simulink model "NR_PDSCH_LinkLevel_Sim"  (R2026a)
settings: Solver=FixedStepDiscrete  StopTime=59  FixedStep=1
InitFcn:
  | addpath(genpath(pwd));
  | if exist('set_sim_profile.m','file'); set_sim_profile('massive'); end
  | cfg = config();
  | assert(cfg.nTx==64 && cfg.nRx==8 && cfg.nLayers==4, ...
  |     'This 64x8 bench needs the massive profile: run set_sim_profile(''massive'')');
  | rng(cfg.randomSeed);
  | run_verification_gates(cfg);   % gates before results
StopFcn:
  | ber = sum(log_bitErrors)/sum(log_nBits);
  | bler = mean(log_blockError);
  | fprintf('\n=== Simulink run aggregate (one SNR point) ===\n');
  | fprintf('BER  = %.5g\nBLER = %.4g\nEVM  = %.4g %%\nNMSE = %.5g\nCapacity = %.4g bit/s/Hz\n', ...
  |     ber, bler, 100*mean(log_evm), mean(log_nmse), mean(log_capacity));
undefined symbols (not defined in the file or in its folder): DiscIntNeverNeededParam
Description:
  | PDSCH-oriented 64x8 Massive MIMO-OFDM link-level test bench, four spatial
  | layers with wideband SVD eigen-beamforming, 144 active subcarriers, 14 OFDM
  | symbols per frame, flat Rayleigh channel. One Monte Carlo frame per step;
  | sixty steps reproduce one SNR point of the massive grid. Every block calls
  | the verified MATLAB chain through thin sl_*.m wrappers; the InitFcn selects
  | the massive profile and runs the verification gates before the first step.
  | Signal dimensions are fixed inside the blocks; rebuilding with
  | build_nr_pdsch_simulink regenerates them from config.m.
settings Model: Creator=mokle  LastModifiedBy=mokle

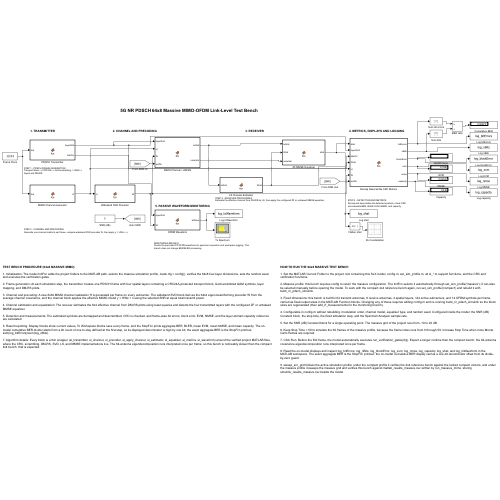
[thumbnail: Simulink's stored preview of the top-level diagram]
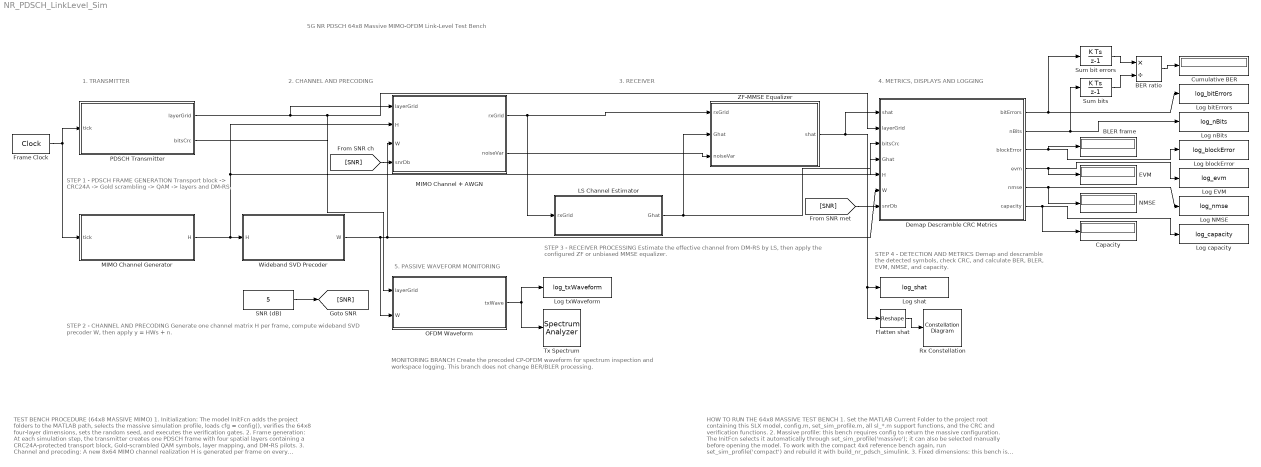
== system NR_PDSCH_LinkLevel_Sim ==
  note: 5G NR PDSCH 64x8 Massive MIMO-OFDM Link-Level Test Bench
  note: 1. TRANSMITTER
  note: 2. CHANNEL AND PRECODING
  note: 3. RECEIVER
  note: 4. METRICS, DISPLAYS AND LOGGING
  note: 5. PASSIVE WAVEFORM MONITORING
  note: STEP 1 - PDSCH FRAME GENERATION
      | Transport block -> CRC24A -> Gold scrambling -> QAM -> layers and DM-RS.
  note: STEP 2 - CHANNEL AND PRECODING
      | Generate one channel matrix H per frame, compute wideband SVD precoder W, then apply y = HWs + n.
  note: STEP 3 - RECEIVER PROCESSING
      | Estimate the effective channel from DM-RS by LS, then apply the configured ZF or unbiased MMSE equalizer.
  note: STEP 4 - DETECTION AND METRICS
      | Demap and descramble the detected symbols, check CRC, and calculate BER, BLER, EVM, NMSE, and capacity.
  note: MONITORING BRANCH
      | Create the precoded CP-OFDM waveform for spectrum inspection and workspace logging. This branch does not change BER/BLER processing.
  note: TEST BENCH PROCEDURE (64x8 MASSIVE MIMO)
      |
      | 1. Initialization: The model InitFcn adds the project folders to the MATLAB path, selects the massive simulation profile, loads cfg = config(), verifies the 64x8 four-layer dimensions, sets the random seed, and executes the verification gates.
      |
      | 2. Frame generation: At each simulation step, the transmitter creates one PDSCH frame with four spatial layers containing a CRC24A-protected transport block, Gold-scrambled QAM symbols, layer mapping, and DM-RS pilots.
      |
      | 3. Channel and precoding: A new 8x64 MIMO channel realization H is generated per frame on every subcarrier. The wideband SVD block derives the 64x4 eigen-beamforming precoder W from the average channel covariance, and the channel block applies the effective MIMO model y = HWs + n using the selected SNR at equal total transmit power.
      |
      | 4. Channel estimation and equalization: The receiver estimates the 8x4 effective channel from DM-RS pilots using least squares and detects the four transmitted layers with the configured ZF or unbiased MMSE equalizer.
      |
      | 5. Detection and measurements: The estimated symbols are demapped and descrambled, CRC is checked, and frame-wise bit errors, block error, EVM, NMSE, and the layer-domain capacity reference are calculated.
      |
      | 6. Result reporting: Display blocks show current values, To Workspace blocks save every frame, and the StopFcn prints aggregate BER, BLER, mean EVM, mean NMSE, and mean capacity. The on-model cumulative BER divider starts from a bit count of one to stay defined at the first step, so its displayed denominator is high by one bit; the exact aggregate BER is the StopFcn printout, sum(log_bitErrors)/sum(log_nBits).
      |
      | 7. Algorithm details: Every block is a thin wrapper (sl_transmitter, sl_channel, sl_precoder, sl_apply_channel, sl_estimator, sl_equalizer, sl_metrics, sl_waveform) around the verified project MATLAB files, where the CRC, scrambling, DM-RS, SVD, LS, and MMSE implementations live. The 64-antenna eigendecomposition runs interpreted once per frame, so this bench is noticeably slower than the compact 4x4 bench; that is expected.
  note: HOW TO RUN THE 64x8 MASSIVE TEST BENCH
      |
      | 1. Set the MATLAB Current Folder to the project root containing this SLX model, config.m, set_sim_profile.m, all sl_*.m support functions, and the CRC and verification functions.
      |
      | 2. Massive profile: this bench requires config to return the massive configuration. The InitFcn selects it automatically through set_sim_profile('massive'); it can also be selected manually before opening the model. To work with the compact 4x4 reference bench again, run set_sim_profile('compact') and rebuild it with build_nr_pdsch_simulink.
      |
      | 3. Fixed dimensions: this bench is built for 64 transmit antennas, 8 receive antennas, 4 spatial layers, 144 active subcarriers, and 14 OFDM symbols per frame, carried as fixed output sizes in the MATLAB Function blocks. Changing any of these requires editing config.m and re-running build_nr_pdsch_simulink so the block sizes are regenerated (then add_rf_measurements for the monitoring branch).
      |
      | 4. Configurable in config.m without rebuilding: modulation order, channel model, equalizer type, and random seed. Configured inside the model: the SNR (dB) Constant block, the stop time, the fixed simulation step, and the Spectrum Analyzer sample rate.
      |
      | 5. Set the SNR (dB) Constant block for a single operating point. The massive grid of the project runs from -10 to 20 dB.
      |
      | 6. Keep Stop Time = 59 to simulate the 60 frames of the massive profile, because the frame index runs from 0 through 59. Increase Stop Time when more Monte Carlo frames are required.
      |
      | 7. Click Run. Before the first frame, the model automatically executes run_verification_gates(cfg). Expect a longer runtime than the compact bench: the 64-antenna covariance eigendecomposition runs interpreted once per frame.
      |
      | 8. Read the on-model displays and inspect log_bitErrors, log_nBits, log_blockError, log_evm, log_nmse, log_capacity, log_shat, and log_txWaveform in the MATLAB workspace. The exact aggregate BER is the StopFcn printout; the on-model cumulative BER display carries a one-bit denominator offset from its divide-by-zero guard.
      |
      | 9. sweep_snr_grid follows the active simulation profile: under the compact profile it verifies the 4x4 reference bench against the locked compact vectors, and under the massive profile it sweeps the massive grid and verifies this bench against matlab_results_massive.csv written by run_massive_mimo, storing simulink_results_massive.csv beside the model.
  BER ratio : Product  Inputs=*/
  BLER frame : Display
  Capacity : Display
  Cumulative BER : Display
  Demap Descramble CRC Metrics : MATLAB Function  TreatAsAtomicUnit=on
  EVM : Display
  Flatten shat : Reshape
  Frame Clock : DigitalClock
  LS Channel Estimator : MATLAB Function  TreatAsAtomicUnit=on
  Log EVM : ToWorkspace  VariableName=log_evm  SampleTime=-1
  Log NMSE : ToWorkspace  VariableName=log_nmse  SampleTime=-1
  Log bitErrors : ToWorkspace  VariableName=log_bitErrors  SampleTime=-1
  Log blockError : ToWorkspace  VariableName=log_blockError  SampleTime=-1
  Log capacity : ToWorkspace  VariableName=log_capacity  SampleTime=-1
  Log nBits : ToWorkspace  VariableName=log_nBits  SampleTime=-1
  Log shat : ToWorkspace  VariableName=log_shat  SampleTime=-1
  Log txWaveform : ToWorkspace  VariableName=log_txWaveform  SampleTime=-1
  MIMO Channel + AWGN : MATLAB Function  TreatAsAtomicUnit=on
  MIMO Channel Generator : MATLAB Function  TreatAsAtomicUnit=on
  NMSE : Display
  OFDM Waveform : MATLAB Function  TreatAsAtomicUnit=on
  PDSCH Transmitter : MATLAB Function  TreatAsAtomicUnit=on
  Rx Constellation : ConstellationDiagram  WindowPosition=[3047.000000,241.000000,600.000000,671.000000,]  ScopeFrameLocation=window  ReferenceConstellation=[-0.948683-0.948683i -0.948683-0.316228i -0.948683+0.316228i -0.948683+0.948683i -0.316228-0.948683i -0.316228-0.316228i -0.316228+0.316228i -0.316228+0.948683i 0.316228-0.948683i 0.316228-0.316228i 0.316228+0.316228i 0.316228+0.948683i 0.948683-0.948683i 0.948683-0.316228i 0.948683+0.316228i 0.948683+0.948683i]
  SNR (dB) : Constant  Value=5  SampleTime=1
  Sum bit errors : DiscreteIntegrator  ICPrevOutput=DiscIntNeverNeededParam  ICPrevScaledInput=DiscIntNeverNeededParam
  Sum bits : DiscreteIntegrator  InitialCondition=1  ICPrevOutput=DiscIntNeverNeededParam  ICPrevScaledInput=DiscIntNeverNeededParam
  Tx Spectrum : SpectrumAnalyzer  WindowPosition=[2247.000000,243.000000,800.000000,668.000000,]  ScopeFrameLocation=window  SampleRateSource=Property  SampleRate=7680000  WindowInvariantSamplesPerUpdate=on  YLimits=[-50.9635 -3.836]
  Wideband SVD Precoder : MATLAB Function  TreatAsAtomicUnit=on
  ZF-MMSE Equalizer : MATLAB Function  TreatAsAtomicUnit=on
  wires:
  Frame Clock/1 -> PDSCH Transmitter/1(tick), MIMO Channel Generator/1(tick)
  SNR (dB)/1 -> [SNR]
  PDSCH Transmitter/1(layerGrid) -> Demap Descramble CRC Metrics/2(layerGrid), OFDM Waveform/1(layerGrid), MIMO Channel + AWGN/1(layerGrid)
  MIMO Channel Generator/1(H) -> MIMO Channel + AWGN/2(H), Demap Descramble CRC Metrics/5(H), Wideband SVD Precoder/1(H)
  Wideband SVD Precoder/1(W) -> MIMO Channel + AWGN/3(W), Demap Descramble CRC Metrics/6(W), OFDM Waveform/2(W)
  [SNR] -> MIMO Channel + AWGN/4(snrDb)
  MIMO Channel + AWGN/1(rxGrid) -> LS Channel Estimator/1(rxGrid), ZF-MMSE Equalizer/1(rxGrid)
  LS Channel Estimator/1(Ghat) -> ZF-MMSE Equalizer/2(Ghat), Demap Descramble CRC Metrics/4(Ghat)
  MIMO Channel + AWGN/2(noiseVar) -> ZF-MMSE Equalizer/3(noiseVar)
  ZF-MMSE Equalizer/1(shat) -> Log shat/1, Flatten shat/1, Demap Descramble CRC Metrics/1(shat)
  PDSCH Transmitter/2(bitsCrc) -> Demap Descramble CRC Metrics/3(bitsCrc)
  [SNR] -> Demap Descramble CRC Metrics/7(snrDb)
  Demap Descramble CRC Metrics/1(bitErrors) -> Sum bit errors/1, Log bitErrors/1
  Demap Descramble CRC Metrics/2(nBits) -> Sum bits/1, Log nBits/1
  Sum bit errors/1 -> BER ratio/1
  Sum bits/1 -> BER ratio/2
  BER ratio/1 -> Cumulative BER/1
  Demap Descramble CRC Metrics/3(blockError) -> BLER frame/1, Log blockError/1
  Demap Descramble CRC Metrics/4(evm) -> EVM/1, Log EVM/1
  Demap Descramble CRC Metrics/5(nmse) -> NMSE/1, Log NMSE/1
  Demap Descramble CRC Metrics/6(capacity) -> Capacity/1, Log capacity/1
  OFDM Waveform/1(txWave) -> Log txWaveform/1, Tx Spectrum/1
  Flatten shat/1 -> Rx Constellation/1

== matlab function NR_PDSCH_LinkLevel_Sim/MIMO Channel Generator ==
  data: tick input; H output
function H = fcn(tick) %#ok<INUSD>
% generate_channel: one realization per frame (AWGN/Rayleigh/Rician/TDL)
coder.extrinsic('sl_channel');
H = complex(zeros(144,8,64));
H = sl_channel(tick);

== matlab function NR_PDSCH_LinkLevel_Sim/PDSCH Transmitter ==
  data: tick input; layerGrid output; bitsCrc output
function [layerGrid, bitsCrc] = fcn(tick) %#ok<INUSD>
% build_frame: TB -> CRC24A -> Gold scrambling -> QAM -> layers + DM-RS
coder.extrinsic('sl_transmitter');
layerGrid = complex(zeros(14,144,4));
bitsCrc = zeros(27648,1);
[layerGrid, bitsCrc] = sl_transmitter(tick);

== matlab function NR_PDSCH_LinkLevel_Sim/Wideband SVD Precoder ==
  data: H input; W output
function W = fcn(H)
% compute_precoder: wideband eigenbeamforming, eq. (31)
coder.extrinsic('sl_precoder');
W = complex(zeros(64,4));
W = sl_precoder(H);

== matlab function NR_PDSCH_LinkLevel_Sim/MIMO Channel + AWGN ==
  data: layerGrid input; rxGrid output; H input; W input; snrDb input; noiseVar output
function [rxGrid, noiseVar] = fcn(layerGrid, H, W, snrDb)
% apply_mimo_channel: y = HWs + n, eq. (34), total-transmit-SNR noise
coder.extrinsic('sl_apply_channel');
rxGrid = complex(zeros(14,144,8));
noiseVar = 0;
[rxGrid, noiseVar] = sl_apply_channel(layerGrid, H, W, snrDb);

== matlab function NR_PDSCH_LinkLevel_Sim/LS Channel Estimator ==
  data: rxGrid input; Ghat output
function Ghat = fcn(rxGrid)
% estimate_effective_channel_ls: LS on DM-RS, eq. (65)
coder.extrinsic('sl_estimator');
Ghat = complex(zeros(144,8,4));
Ghat = sl_estimator(rxGrid);

== matlab function NR_PDSCH_LinkLevel_Sim/ZF-MMSE Equalizer ==
  data: rxGrid input; shat output; Ghat input; noiseVar input
function shat = fcn(rxGrid, Ghat, noiseVar)
% equalize_mimo: ZF eq. (38) or unbiased MMSE eq. (39), per config.m
coder.extrinsic('sl_equalizer');
shat = complex(zeros(1728,4));
shat = sl_equalizer(rxGrid, Ghat, noiseVar);

== matlab function NR_PDSCH_LinkLevel_Sim/Demap Descramble CRC Metrics ==
  data: shat input; bitErrors output; layerGrid input; bitsCrc input; Ghat input; H input; W input; snrDb input; nBits output; blockError output; evm output; nmse output; capacity output
function [bitErrors, nBits, blockError, evm, nmse, capacity] = fcn(shat, layerGrid, bitsCrc, Ghat, H, W, snrDb)
% compute_frame_metrics: BER (41), BLER (42), EVM (43), NMSE (78), C (110)
coder.extrinsic('sl_metrics');
bitErrors = 0; nBits = 0; blockError = 0; evm = 0; nmse = 0; capacity = 0;
[bitErrors, nBits, blockError, evm, nmse, capacity] = sl_metrics(shat, layerGrid, bitsCrc, Ghat, H, W, snrDb);

== matlab function NR_PDSCH_LinkLevel_Sim/OFDM Waveform ==
  data: layerGrid input; txWave output; W input
function txWave = fcn(layerGrid, W)
% ofdm_modulate on the precoded grid: time-domain CP-OFDM waveform
coder.extrinsic('sl_waveform');
txWave = complex(zeros(3836,64));
txWave = sl_waveform(layerGrid, W);
